simulink model "day05p2"  (R2026a)
settings: Solver=VariableStepAuto  StopTime=inf
undefined symbols (not defined in the file): DiscIntNeverNeededParam
libraries: simulink x1, dspstat3 x1
settings Model: Creator=pete  LastModifiedBy=pete

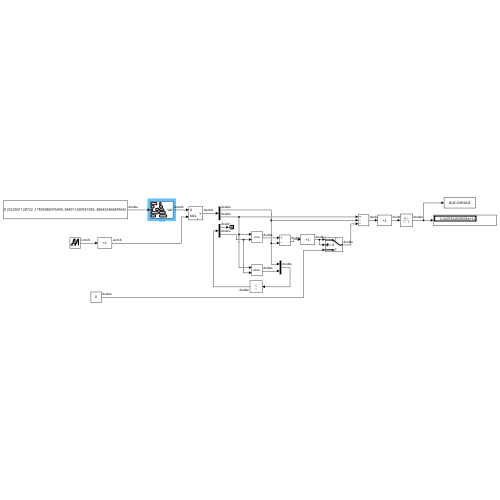
[thumbnail: Simulink's stored preview of the top-level diagram]
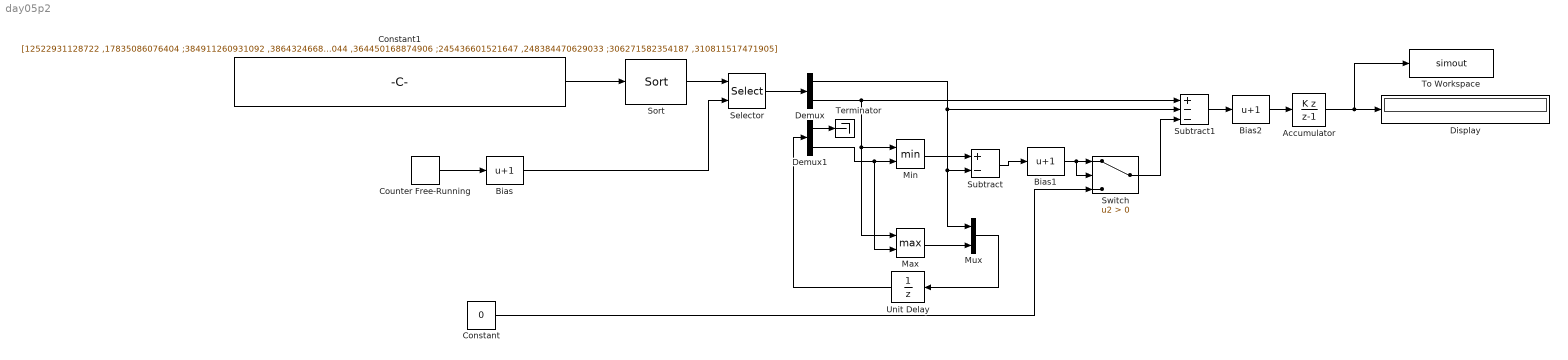
== system day05p2 ==
  Accumulator : DiscreteIntegrator  IntegratorMethod=Accumulation: Backward Euler  SampleTime=-1  ICPrevOutput=DiscIntNeverNeededParam  ICPrevScaledInput=DiscIntNeverNeededParam
  Bias : Bias  Bias=1  SaturateOnIntegerOverflow=off
  Bias1 : Bias  Bias=1  SaturateOnIntegerOverflow=off
  Bias2 : Bias  Bias=1  SaturateOnIntegerOverflow=off
  Constant : Constant  Value=0
  Constant1 : Constant  Value=[12522931128722 ,17835086076404 ;384911260931092 ,386432466839642 ;365270830395340 ,365971888864203 ;335965656565989 ,338385913690745 ;344444810072307 ,346735887081443 ;517987696536841 ,521724333531860 ;196616352567120 ,198928304566201 ;153221685952097 ,153755911901684 ;534143330816947 ,538769212631051 ;182468249249495 ,187418315879123 ;43144734757249 ,43577434669619 ;96196757409900 ,97842950488786 ;363494394902627 ,364104305337144 ;323545976685828 ,328381600514770 ;466365467671134 ,468743303650602 ;33404129353255 ,39408988150975 ;211180171561966 ,213266641390525 ;205211856590532 ,208854464057250 ;415721649347453 ,418094982195439 ;254204192528400 ,260697055883379 ;367873153721253 ,368016310110182 ;42442739340807 ,43144734757249 ;219253350919822 ,221053580591060 ;43577434669619 ,44073101250782 ;525856347827494 ,531481049142511 ;81886655886201 ,83640283511310 ;474954993123386 ,477586533724840 ;534143330816947 ,538769212631051 ;384131201179338 ,385573225027240 ;447749683702651 ,450391818945542 ;85178915987694 ,86897282432691 ;561314402345593 ,561467755875554 ;296769207971316 ,301237803346584 ;369236321979649 ,369557094002763 ;413858958468963 ,420801621640271 ;561803939480482 ,562405452295386 ;346735887081444 ,349433264449869 ;123748864457105 ,130040447979081 ;561803939480482 ,562107381752145 ;114098974651581 ,117409557005873 ;161894929122853 ,169121277933470 ;555736617876554 ,556241804964044 ;156239660754332 ,156389455668514 ;388621919665330 ,389858455161035 ;42139357182737 ,42831565435472 ;558528122612271 ,558770826138679 ;324617547245941 ,329941639145753 ;12522931128722 ,15293222563191 ;102614529425745 ,108649683941988 ;213679961337545 ,215123497855253 ;135857961289697 ,138332328930082 ;236624785606395 ,239092217398990 ;499835849397777 ,499835849397777 ;363791433835044 ,364324982892722 ;172738985769002 ,177518418069748 ;558344787311370 ,558528122612271 ;353084605827971 ,360393800154139 ;365507310440850 ,366325903877499 ;335965656565988 ,335965656565988 ;453698284380589 ,453698284380589 ;367539770344201 ,367873153721253 ;462921956273886 ,465397950365611 ;312484362041096 ,316126210732700 ;382248542386326 ,383628575706719 ;133582436738612 ,135857961289695 ;42139357182737 ,42442739340807 ;192126052775114 ,198928304566201 ;389372362148921 ,390742801075286 ;387680474913661 ,389091391390315 ;372646859877968 ,380918608719276 ;560362765835933 ,561079617055758 ;83154152608943 ,84488314861730 ;364324982892722 ,364798016791139 ;437450269240455 ,441761281682837 ;42442739340807 ,42642042567067 ;372646859877968 ,372646859877968 ;40597746185338 ,41317963814134 ;558988099077195 ,559219039863863 ;153917561839048 ,154491257171632 ;385868222920649 ,387289408618892 ;242127501119589 ,251045924420956 ;368314044607872 ,368593252171558 ;43577434669619 ,43816326444333 ;361949183562057 ,362490604548609 ;544538825545876 ,551850196688314 ;153755911901684 ,154120537338723 ;515031870020511 ,517987696536840 ;393272531621358 ,401459444239884 ;214685522373596 ,216529423211432 ;383024284949594 ,384609577190183 ;367324717063976 ,367873153721253 ;91926437467533 ,96196757409899 ;495241741768371 ,499835849397777 ;80553444766235 ,82489739224950 ;46198548440032 ,46384786108890 ;54633221641607 ,58320458217135 ;153755911901684 ,153917561839048 ;490051825862601 ,490051825862601 ;154632322317176 ,154944463744259 ;558528122612271 ,558770826138679 ;40597746185338 ,41047522349447 ;215962563233885 ,217313482241748 ;54633221641607 ,58320458217135 ;312484362041096 ,319503879582902 ;444366237309702 ,450391818945542 ;365971888864203 ,366325903877499 ;212321963245239 ,214162860750709 ;7840509071694 ,7840509071694 ;524948588738162 ,529035212328467 ;154120537338723 ,154944463744259 ;158696163972883 ,159423257729154 ;260697055883379 ,260697055883379 ;45962138792094 ,46582719251296 ;40824152734012 ,41047522349447 ;123748864457104 ,123748864457104 ;386790280879461 ,388022546024271 ;31928040599678 ,37248039217929 ;216830351007525 ,218484949158117 ;142276088645327 ,147302961991049 ...(+2207 chars)]
  Counter Free-Running : simulink/Sources/Counter Free-Running  NumBits=16  tsamp=-1
  Demux : Demux  Outputs=2
  Demux1 : Demux  Outputs=2
  Display : Display
  Max : MinMax  Function=max  Inputs=2
  Min : MinMax  Inputs=2
  Mux : Mux  Inputs=2
  Selector : Selector  NumberOfDimensions=2  InputPortWidth=3  IndexOptions=Index vector (port),Index vector (dialog)  Indices=[1 3],[1 2]  OutputSizes=1,1
  Sort : dspstat3/Sort  otype=Value  dir=Ascending  sortAlg=Quick sort  roundingMode=Floor  overflowMode=off  accumDataTypeStr=Inherit: Same as product output  accumLastDataTypeStr=Inherit: Same as product output
  Subtract : Sum  Inputs=+-
  Subtract1 : Sum  Inputs=+--
  Switch : Switch  Criteria=u2 > Threshold  SaturateOnIntegerOverflow=off  InputSameDT=off
  Terminator : Terminator
  To Workspace : ToWorkspace  VariableName=simout  SaveFormat=Timeseries  SampleTime=-1
  Unit Delay : UnitDelay  SampleTime=-1
  wires:
  Counter Free-Running/1 -> Bias/1
  Bias/1 -> Selector/2
  Sort/1 -> Selector/1
  Selector/1 -> Demux/1
  Constant1/1 -> Sort/1
  Min/1 -> Subtract/1
  Demux1/2 -> Max/2, Min/2
  Demux/2 -> Subtract1/1, Max/1, Min/1
  Demux1/1 -> Terminator/1
  Demux/1 -> Subtract1/2, Mux/1, Subtract/2
  Max/1 -> Mux/2
  Subtract/1 -> Bias1/1
  Bias1/1 -> Switch/2, Switch/1
  Constant/1 -> Switch/3
  Switch/1 -> Subtract1/3
  Subtract1/1 -> Bias2/1
  Bias2/1 -> Accumulator/1
  Accumulator/1 -> To Workspace/1, Display/1
  Mux/1 -> Unit Delay/1
  Unit Delay/1 -> Demux1/1
